simulink model "tvcrocketsim_rev2"  (R2022a)
settings: Solver=VariableStepAuto  StartTime=0.0  StopTime=10.0  RelTol=1e-3
undefined symbols (not defined in the file): X
libraries: simulink_extras x2, slpidlib x1, shared3dof x1
settings Model: Creator=elija  LastModifiedBy=elija

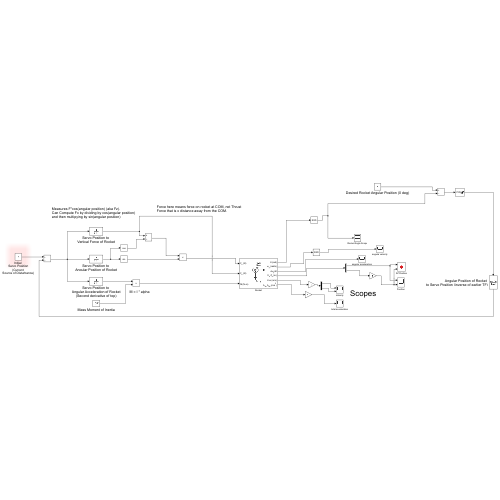
[thumbnail: Simulink's stored preview of the top-level diagram]
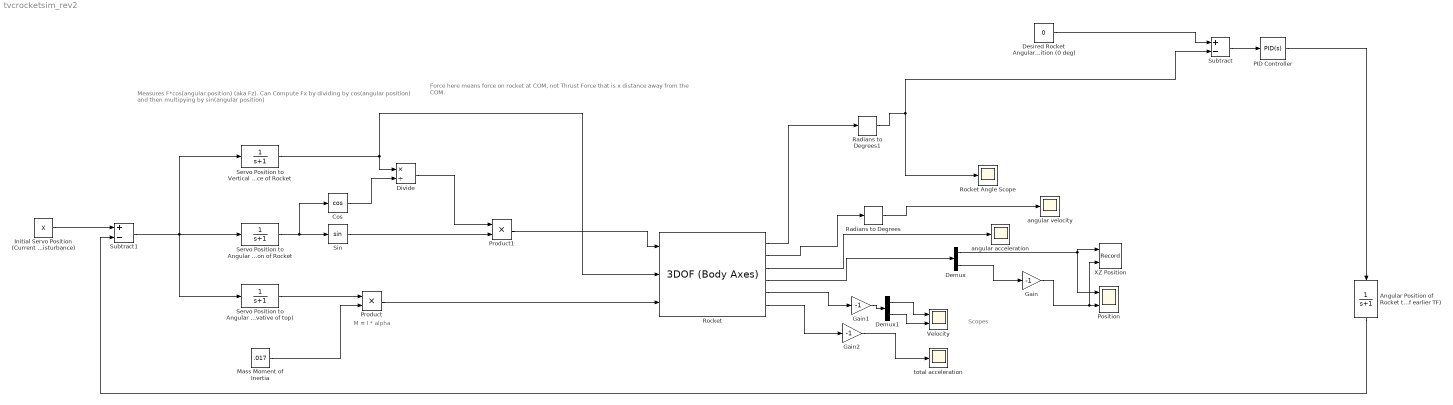
== system tvcrocketsim_rev2 ==
  note: Force here means force on rocket at COM, not Thrust Force that is x distance away from the COM.
  note: Scopes
  note: Measures F*cos(angular position) (aka Fz).
      | Can Compute Fx by dividing by cos(angular position) and then multipying by sin(angular position)
  note: M = I * alpha
  Angular Position of Rocket to Servo Position (inverse of earlier TF) : TransferFcn  Denominator=[1 1]
  Cos : Trigonometry  Operator=cos
  Demux : Demux  Outputs=2
  Demux1 : Demux  Outputs=2
  Desired Rocket Angular Position (0 deg) : Constant  Value=0
  Divide : Product  Inputs=*/
  Gain : Gain  Gain=-1
  Gain1 : Gain  Gain=-1
  Gain2 : Gain  Gain=-1
  Initial Servo Position (Current Source of Disturbance) : Constant  Value=X
  Mass Moment of Inertia : Constant  Value=.017
  PID Controller : slpidlib/PID Controller  Controller=PID  Form=Parallel  TimeDomain=Continuous-time  UseExternalTs=off  SampleTime=-1  IntegratorMethod=Forward Euler  FilterMethod=Forward Euler  ControllerParametersSource=internal  P=.35  I=0  UseKiTs=off  D=.08  N=100  UseFilter=on  TunerSelectOption=Frequency Response Based  InitialConditionSource=internal  InitialConditionForIntegrator=0  InitialConditionForFilter=0  DifferentiatorICPrevScaledInput=0  ExternalReset=none  TrackingMode=off  Kt=1  LimitOutput=on  SatLimitsSource=internal  UpperSaturationLimit=5  LowerSaturationLimit=-5  LinearizeAsGain=on  AntiWindupMode=none  Kb=1  POutMin=[]  POutMax=[]  IOutMin=[]  IOutMax=[]  DOutMin=[]  DOutMax=[]  NOutMin=[]  NOutMax=[]  SumOutMin=[]  SumOutMax=[]  SaturationOutMin=[]  SaturationOutMax=[]  PParamMin=[]  PParamMax=[]  IParamMin=[]  IParamMax=[]  DParamMin=[]  DParamMax=[]  NParamMin=[]  NParamMax=[]  KbParamMin=[]  KbParamMax=[]  KtParamMin=[]  KtParamMax=[]  KbOutMin=[]  KbOutMax=[]  KtOutMin=[]  KtOutMax=[]  IntegratorOutMin=[]  IntegratorOutMax=[]  FilterOutMin=[]  FilterOutMax=[]  SumI1OutMin=[]  SumI1OutMax=[]  SumI2OutMin=[]  SumI2OutMax=[]  SumI3OutMin=[]  SumI3OutMax=[]  SumI4OutMin=[]  SumI4OutMax=[]  SumDOutMin=[]  SumDOutMax=[]  DifferentiatorOutMin=[]  DifferentiatorOutMax=[]  FilterDiffOutCoefMin=[]  FilterDiffOutCoefMax=[]  ReciprocalOutMin=[]  ReciprocalOutMax=[]  SumDenOutMin=[]  SumDenOutMax=[]  SumNumOutMin=[]  SumNumOutMax=[]  DivideOutMin=[]  DivideOutMax=[]  UdiffTsProdOutMin=[]  UdiffTsProdOutMax=[]  NTsProdOutMin=[]  NTsProdOutMax=[]  UintegralTsProdOutMin=[]  UintegralTsProdOutMax=[]  UngainTsProdOutMin=[]  UngainTsProdOutMax=[]  IntegratorContinuousStateAttributes=''  IntegratorStateMustResolveToSignalObject=off  IntegratorRTWStateStorageClass=Auto  FilterContinuousStateAttributes=''  FilterStateMustResolveToSignalObject=off  FilterRTWStateStorageClass=Auto  ParallelPVariant=InternalParameters  IdealPVariant=Disabled  IVariant=InternalParameters  DVariant=InternalParameters  IntegratorVariant=Continuous  SatVariant=Enabled  AWVariant=Passthrough  PCopyVariant=Disabled  TRVariant=Disabled  FdbkBlocksVariant=Forward  IdealPFdbkVariant=Disabled  SatFdbkVariant=Disabled  DerivativeFilterVariant=ContFilter  NVariant=InternalParameters  NCopyVariant=Disabled  FilterICVariant=InternalICsFilter  IntegratorICVariant=InternalICs  ExternalResetVariant=Disabled  TRSumVariant=Passthrough  SumFdbkVariant=Disabled  SumVariant=Sum_PID  TsampFilterVariant=InternalTs  TsampNgainVariant=Passthrough  TsampIntegralVariant=Passthrough  ExternalSaturationOutDataTypeStr=Inherit: Same as second input  aMode=0
  Position : Scope  NumInputPorts=2
  Product : Product
  Product1 : Product
  Radians to Degrees : simulink_extras/Transformations/Radians to Degrees
  Radians to Degrees1 : simulink_extras/Transformations/Radians to Degrees
  Rocket : shared3dof/3DOF (Body Axes)  units=Metric (MKS)  mtype=Fixed  v_ini=0  theta_ini=0  alpha_ini=3  pos_ini=[0 0]  q_ini=0  mass=.805  mass_e=0.5  mass_f=3.0  Iyy=.017  Iyy_e=0.5  Iyy_f=3.0  g_in=Internal  g=9.81  vre_flag=on  abi_flag=off  aMode=0  vel_statename=''  theta_statename=''  pos_statename=''  q_statename=''  mass_statename=''
      settings: SourceProductBaseCode=AE,PW,DR,MT,VE
  Rocket Angle Scope : Scope
  Servo Position to Angular Acceleration of Rocket (Second derivative of top) : TransferFcn  Denominator=[1 1]
  Servo Position to Angular Position of Rocket : TransferFcn  Denominator=[1 1]
  Servo Position to Vertical Force of Rocket : TransferFcn  Denominator=[1 1]
  Sin : Trigonometry
  Subtract : Sum  Inputs=+-
  Subtract1 : Sum  Inputs=+-
  Velocity : Scope  NumInputPorts=2
  XZ Position : Record  FileSettingsInternal="{\"entries\":[{\"content\":{\"excelSettings\":{\"content\":{},\"type\":\"Streamout.ExcelSettings\"}},\"type\":\"Streamout.FileSettingStorage\",\"uuid\":\"68ac2f9b-6c08-4650-a068-6719ff741537\"}],\"packageUris\":[\"http://schema.mathworks.com/mf0/streamout_blocks/R2020a\"],\"version\":\"1.0\"}"  Layout=[1 1]  SignalsInternal="{\"entries\":[{\"content\":{\"signals\":[{\"content\":{\"blockPath\":[\"untitled/XZ Position\"],\"channel\":[],\"dimensions\":[1],\"domain\":\"untitled/XZ Position\",\"lineColor\":\"#a2142f\",\"plots\":[1],\"port\":1,\"sid\":[],\"signalID\":48,\"signalName\":\"XY Graph:1\"},\"type\":\"RecordBlkView.Signal\",\"uuid\":\"8732acea-ac2b-489a-a7ed-ed1c92d07ca7\"},{\"content\":{\"blockPath\":[\"untitled/XZ Position\"],\"channel\":[],\"dimensions\":[1],\"domain\":\"untitled/XZ Position\",\"lineColor\":\"#139fff\",\"plots\":[1],\"port\":2,\"sid\":[],\"signalID\":51,\"signalName\":\"XY Graph:2\"},\"type\":\"RecordBlkView.Signal\",\"uuid\":\"a78a397f-30f0-48f1-aba9-68f0534c1a87\"}]},\"type\":\"RecordBlkView.InputSignals\",\"uuid\":\"6d6dc71a-b703-42c9-b069-9ebf1a7cdffc\"}],\"packageUris\":[\"http://schema.mathworks.com/mf0/streamout_blocks/R2020a\"],\"version\":\"1.0\"}"  VisualizationBindings="{\"xyplotplugin\":{\"info\":[{\"series\":[{\"bindingParametersList\":[{\"parameter\":\"X-Axis\",\"signalID\":48,\"signalName\":\"XY Graph:1\"},{\"parameter\":\"Y-Axis\",\"signalID\":51,\"signalName\":\"XY Graph:2\"}],\"seriesID\":62603}],\"subplotID\":1}]}}"  CompatibilityTag=XY  st=-1
  angular acceleration : Scope
  angular velocity : Scope
  total acceleration : Scope
  wires:
  Subtract1/1 -> Servo Position to Vertical Force of Rocket/1, Servo Position to Angular Position of Rocket/1, Servo Position to Angular Acceleration of Rocket (Second derivative of top)/1
  Rocket/3 -> angular acceleration/1
  PID Controller/1 -> Angular Position of Rocket to Servo Position (inverse of earlier TF)/1
  Rocket/2 -> Radians to Degrees/1
  Initial Servo Position (Current Source of Disturbance)/1 -> Subtract1/1
  Desired Rocket Angular Position (0 deg)/1 -> Subtract/1
  Rocket/4 -> Demux/1
  Gain/1 -> XZ Position/2, Position/2
  Radians to Degrees1/1 -> Subtract/2, Rocket Angle Scope/1
  Subtract/1 -> PID Controller/1
  Radians to Degrees/1 -> angular velocity/1
  Demux1/1 -> Velocity/1
  Demux/2 -> Gain/1
  Gain1/1 -> Demux1/1
  Gain2/1 -> total acceleration/1
  Demux1/2 -> Velocity/2
  Rocket/6 -> Gain2/1
  Rocket/1 -> Radians to Degrees1/1
  Rocket/5 -> Gain1/1
  Demux/1 -> XZ Position/1, Position/1
  Servo Position to Angular Acceleration of Rocket (Second derivative of top)/1 -> Product/1
  Mass Moment of Inertia/1 -> Product/2
  Product/1 -> Rocket/3
  Servo Position to Vertical Force of Rocket/1 -> Rocket/2, Divide/1
  Servo Position to Angular Position of Rocket/1 -> Cos/1, Sin/1
  Cos/1 -> Divide/2
  Sin/1 -> Product1/2
  Divide/1 -> Product1/1
  Product1/1 -> Rocket/1
  Angular Position of Rocket to Servo Position (inverse of earlier TF)/1 -> Subtract1/2
